simulink model "lyap_sim"  (Simulink 5.0)
settings: Solver=ode45  SolverMode=SingleTasking  StartTime=0.0  StopTime=80  FixedStep=0.001  RelTol=1e-3
settings Model: LastModifiedBy=Administrator  ExtModeTrigMode=oneshot  ExtModeArmWhenConnect=off  LimitDataPoints=off  BooleanDataType=off

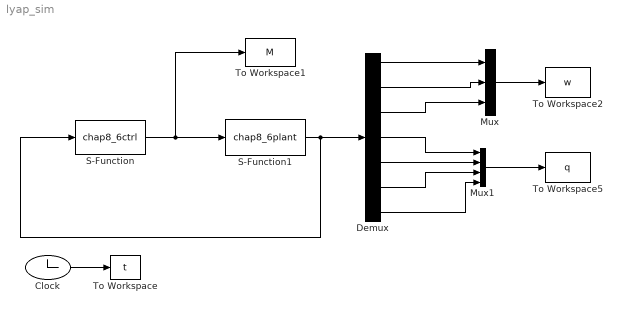
== system lyap_sim ==
  Clock : Clock
  Demux : Demux  Outputs=7
  Mux : Mux  Inputs=3
  Mux1 : Mux
  S-Function : S-Function  FunctionName=chap8_6ctrl
  S-Function1 : S-Function  FunctionName=chap8_6plant
  To Workspace : ToWorkspace  VariableName=t  SampleTime=-1  SaveFormat=Array
  To Workspace1 : ToWorkspace  VariableName=M  SampleTime=-1  SaveFormat=Array
  To Workspace2 : ToWorkspace  VariableName=w  SampleTime=-1  SaveFormat=Array
  To Workspace5 : ToWorkspace  VariableName=q  SampleTime=-1  SaveFormat=Array
  wires:
  S-Function/1 -> S-Function1/1, To Workspace1/1
  S-Function1/1 -> S-Function/1, Demux/1
  Demux/1 -> Mux/1
  Demux/2 -> Mux/2
  Demux/3 -> Mux/3
  Mux/1 -> To Workspace2/1
  Mux1/1 -> To Workspace5/1
  Demux/4 -> Mux1/1
  Demux/5 -> Mux1/2
  Demux/6 -> Mux1/3
  Demux/7 -> Mux1/4
  Clock/1 -> To Workspace/1
